simulink model "randomControllerSim2OLD"  (R2015a)
settings: Solver=ode45  SolverMode=SingleTasking  StartTime=0.0  StopTime=1.5  RelTol=1e-3
values from neighbouring files (symbols this model uses):
  B_f = 7.4e-3    (= 0.0074)    [randomController.m]
  B_w = 17.03e-6    (= 1.703e-05)    [randomController.m]
  g = 9.82    [randomController.m]
  J_f = 5.6e-3    (= 0.0056)    [randomController.m]
  J_w = 0.601e-3    (= 0.000601)    [randomController.m]
  l_f = 0.08498    [randomController.m]
  l_w = 0.093    [randomController.m]
  m_f = 0.77-m_w    (= 0.548)    [randomController.m]
  m_w = 0.222    [randomController.m]
undefined symbols (not defined in the file or in its folder): disturb, t_dist
settings Model: CovSFcnEnable=off  Creator=USUARIO  LastModifiedBy=USUARIO
settings OptimizationCC: BlockReduction=off  BooleanDataType=off
settings DebuggingCC: SaveWithParameterizedLinksMsg=none  UnderspecifiedInitializationDetection=Classic  MergeDetectMultiDrivingBlocksExec=none  SignalResolutionControl=TryResolveAllWithWarning
settings HardwareCC: TargetUnknown=on

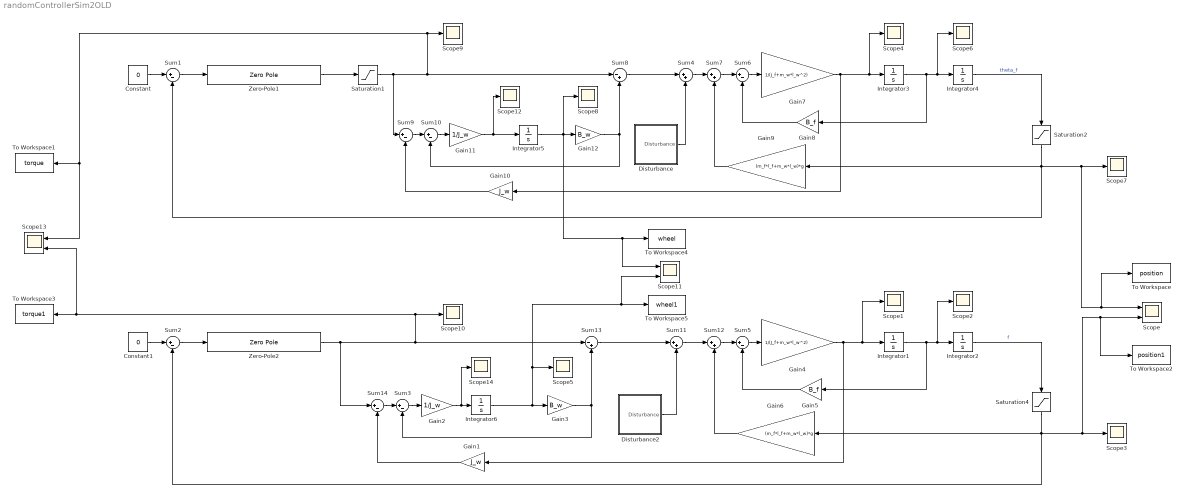
== system randomControllerSim2OLD ==
  Constant : Constant  Value=0
  Constant1 : Constant  Value=0
  Disturbance : Subsystem
  Disturbance2 : Subsystem
  Gain1 : Gain  Gain=J_w
  Gain10 : Gain  Gain=J_w
  Gain11 : Gain  Gain=1/J_w
  Gain12 : Gain  Gain=B_w
  Gain2 : Gain  Gain=1/J_w
  Gain3 : Gain  Gain=B_w
  Gain4 : Gain  Gain=1/(J_f+m_w*l_w^2)
  Gain5 : Gain  Gain=B_f
  Gain6 : Gain  Gain=(m_f*l_f+m_w*l_w)*g
  Gain7 : Gain  Gain=1/(J_f+m_w*l_w^2)
  Gain8 : Gain  Gain=B_f
  Gain9 : Gain  Gain=(m_f*l_f+m_w*l_w)*g
  Integrator{1..6} (6 alike) : Integrator
  Saturation1 : Saturate  UpperLimit=4*0.0335  LowerLimit=-4*0.0335
  Saturation2 : Saturate  UpperLimit=0.85  LowerLimit=-0.72
  Saturation4 : Saturate  UpperLimit=0.85  LowerLimit=-0.72
  Scope : Scope  NumInputPorts=2
      settings: TimeRange=auto  MaxDataPoints=5000  SaveToWorkspace=off  YMin=-0.02803~-5  YMax=0.02788~5  SampleTime=-1
  Scope{1..10,12,14} (12 alike) : Scope
      Scope1 settings: TimeRange=auto  LimitDataPoints=on  MaxDataPoints=5000  SaveToWorkspace=off  YMin=-10  YMax=10  SampleTime=-1  DataFormat=Array
      Scope10 settings: TimeRange=auto  LimitDataPoints=on  MaxDataPoints=5000  SaveToWorkspace=off  SaveName=ScopeData2  YMin=-0.18111  YMax=0.46457  SampleTime=-1  DataFormat=Array
      Scope12 settings: TimeRange=auto  LimitDataPoints=on  MaxDataPoints=5000  SaveToWorkspace=off  SaveName=ScopeData5  YMin=-10  YMax=10  SampleTime=-1  DataFormat=Array
      Scope14 settings: TimeRange=auto  LimitDataPoints=on  MaxDataPoints=5000  SaveToWorkspace=off  SaveName=ScopeData4  YMin=-324.30879  YMax=834.64358  SampleTime=-1  DataFormat=Array
      Scope2 settings: TimeRange=auto  LimitDataPoints=on  MaxDataPoints=5000  SaveToWorkspace=off  SaveName=ScopeData3  YMin=-10  YMax=10  SampleTime=-1  DataFormat=Array
      Scope3 settings: TimeRange=auto  LimitDataPoints=on  MaxDataPoints=5000  SaveToWorkspace=off  SaveName=ScopeData4  YMin=-0.01906  YMax=0.01828  SampleTime=-1  DataFormat=Array
      Scope4 settings: TimeRange=auto  LimitDataPoints=on  MaxDataPoints=5000  SaveToWorkspace=off  SaveName=ScopeData  YMin=-10  YMax=10  SampleTime=-1  DataFormat=Array
      Scope5 settings: TimeRange=auto  LimitDataPoints=on  MaxDataPoints=5000  SaveToWorkspace=off  SaveName=ScopeData5  YMin=-8.89852  YMax=11.79883  SampleTime=-1  DataFormat=Array
      Scope6 settings: TimeRange=auto  LimitDataPoints=on  MaxDataPoints=5000  SaveToWorkspace=off  SaveName=ScopeData  YMin=-10  YMax=10  SampleTime=-1  DataFormat=Array
      Scope7 settings: TimeRange=auto  LimitDataPoints=on  MaxDataPoints=5000  SaveToWorkspace=off  SaveName=ScopeData  YMin=-0.01906  YMax=0.01828  SampleTime=-1  DataFormat=Array
      Scope8 settings: TimeRange=auto  LimitDataPoints=on  MaxDataPoints=5000  SaveToWorkspace=off  SaveName=ScopeData  YMin=-9.64267  YMax=11.88152  SampleTime=-1  DataFormat=Array
      Scope9 settings: TimeRange=auto  LimitDataPoints=on  MaxDataPoints=5000  SaveToWorkspace=off  SaveName=ScopeData  YMin=-0.2195  YMax=0.6355  SampleTime=-1  DataFormat=Array
  Scope11 : Scope  NumInputPorts=2
      settings: TimeRange=auto  MaxDataPoints=5000  SaveToWorkspace=off  YMin=-9.64267~-5  YMax=11.88152~5  SampleTime=-1
  Scope13 : Scope  NumInputPorts=2
      settings: TimeRange=auto  MaxDataPoints=5000  SaveToWorkspace=off  SaveName=ScopeData3  YMin=-0.06395~-5  YMax=0.1859~5  SampleTime=-1
  Sum{1..3,5..6,9..10,14} (8 alike) : Sum  Inputs=|+-
  Sum{4,7,11..12} (4 alike) : Sum  Inputs=|++
  Sum13 : Sum  Inputs=|-+
  Sum8 : Sum  Inputs=|-+
  To Workspace : ToWorkspace  VariableName=position  SaveFormat=Timeseries  SampleTime=-1
  To Workspace1 : ToWorkspace  VariableName=torque  SaveFormat=Timeseries  SampleTime=-1
  To Workspace2 : ToWorkspace  VariableName=position1  SaveFormat=Timeseries  SampleTime=-1
  To Workspace3 : ToWorkspace  VariableName=torque1  SaveFormat=Timeseries  SampleTime=-1
  To Workspace4 : ToWorkspace  VariableName=wheel  SaveFormat=Timeseries  SampleTime=-1
  To Workspace5 : ToWorkspace  VariableName=wheel1  SaveFormat=Timeseries  SampleTime=-1
  Zero-Pole1 : ZeroPole  Zeros=[-9.483 -1.599]  Poles=[-200 -100 5.539]  Gain=[-0.62737*200*100*5.539/9.483/1.599]
  Zero-Pole2 : ZeroPole  Zeros=[-9.483 -1.599]  Poles=[-200 -100 5.539]  Gain=[-0.62737*200*100*5.539/9.483/1.599]
  wires:
  Gain7/1 -> Gain10/1, Scope4/1, Integrator3/1
  Integrator3/1 -> Gain8/1, Scope6/1, Integrator4/1
  Sum6/1 -> Gain7/1
  Sum7/1 -> Sum6/1
  Gain8/1 -> Sum6/2
  Gain9/1 -> Sum7/2
  Sum10/1 -> Gain11/1
  Gain11/1 -> Scope12/1, Integrator5/1
  Gain10/1 -> Sum9/2
  Sum9/1 -> Sum10/1
  Integrator5/1 -> To Workspace4/1, Scope11/1, Scope8/1, Gain12/1
  Gain12/1 -> Sum10/2, Sum8/2
  Sum1/1 -> Zero-Pole1/1
  Constant/1 -> Sum1/1
  Saturation2/1 -> Scope7/1, To Workspace/1, Scope/1, Sum1/2, Gain9/1
  Gain4/1 -> Integrator1/1, Scope1/1, Gain1/1
  Integrator1/1 -> Gain5/1, Scope2/1, Integrator2/1
  Sum5/1 -> Gain4/1
  Sum12/1 -> Sum5/1
  Gain5/1 -> Sum5/2
  Gain6/1 -> Sum12/2
  Sum3/1 -> Gain2/1
  Gain2/1 -> Scope14/1, Integrator6/1
  Gain1/1 -> Sum14/2
  Sum14/1 -> Sum3/1
  Integrator6/1 -> Gain3/1, Scope5/1, To Workspace5/1, Scope11/2
  Gain3/1 -> Sum13/2, Sum3/2
  Integrator2/1 -> Saturation4/1  "f"
  Sum2/1 -> Zero-Pole2/1
  Constant1/1 -> Sum2/1
  Saturation4/1 -> Scope3/1, Scope/2, To Workspace2/1, Sum2/2, Gain6/1
  Zero-Pole2/1 -> Sum13/1, Scope10/1, Scope13/2, To Workspace3/1, Sum14/1
  Saturation1/1 -> Sum8/1, Scope9/1, To Workspace1/1, Scope13/1, Sum9/1
  Zero-Pole1/1 -> Saturation1/1
  Integrator4/1 -> Saturation2/1  "theta_f"
  Disturbance/1(Disturbance) -> Sum4/2
  Sum8/1 -> Sum4/1
  Sum4/1 -> Sum7/1
  Disturbance2/1(Disturbance) -> Sum11/2
  Sum11/1 -> Sum12/1
  Sum13/1 -> Sum11/1

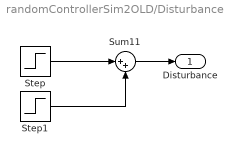
== system randomControllerSim2OLD/Disturbance ==
  Step : Step  Time=0.1  After=disturb  SampleTime=0
  Step1 : Step  Time=0.1+t_dist  After=-disturb  SampleTime=0
  Sum11 : Sum  Inputs=|++
  Disturbance : Outport
  wires:
  Step1/1 -> Sum11/2
  Step/1 -> Sum11/1
  Sum11/1 -> Disturbance/1

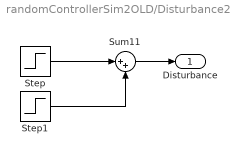
== system randomControllerSim2OLD/Disturbance2 ==
  Step : Step  Time=0.1  After=disturb  SampleTime=0
  Step1 : Step  Time=0.1+t_dist  After=-disturb  SampleTime=0
  Sum11 : Sum  Inputs=|++
  Disturbance : Outport
  wires:
  Sum11/1 -> Disturbance/1
  Step/1 -> Sum11/1
  Step1/1 -> Sum11/2
